simulink model "centroid"  (R2017b)
settings: Solver=VariableStepAuto  StartTime=0.0  StopTime=10.0  RelTol=1e-3
settings Model: Creator=Administrator  LastModifiedBy=Administrator

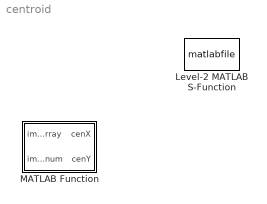
== system centroid ==
  Level-2 MATLAB S-Function : M-S-Function  FunctionName=matlabfile
  MATLAB Function : MATLAB Function  TreatAsAtomicUnit=on

== matlab function centroid/MATLAB Function ==
  data: img_array input; cenX output; img_num input; cenY output
function [cenX,cenY] = cu_cenroid(img_array,img_num)
% 本函数用于计算若干张图像数据的质心位置，图像有先后顺序但无逻辑顺序。
% 本函数是labview 并行计划的第一环
% 本函数必须假设图像矩阵是长宽一致的。

% 第一步，确定图像总矩阵大小
 ROI_size = size(img_array,2);
 mass_array_x = zeros(ROI_size);
 mass_array_y = zeros(ROI_size);
 cenX = zeros(img_num,1);
 cenY = zeros(img_num,1);
 % 第二步，划分成若干图像
 for i = 1:img_num
     img = img_array((1+ROI_size*(i-1)):ROI_size*i,1:ROI_size);
     mass = sum(sum(img));
     for j = 1:ROI_size
         for k  = 1:ROI_size
             mass_array_x(j,k) = img(j,k)* k;
             mass_array_y(j,k) = img(j,k)* j;
         end 
     end
     cenX(i) = sum(sum(mass_array_x))/mass;
     cenY(i) = sum(sum(mass_array_y))/mass;
     
end
